simulink model "rev2_PEM"  (R2024a)
settings: Solver=VariableStepAuto  StartTime=0.0  StopTime=10.0  RelTol=1e-3
libraries: spsParallelRLCBranchLib x3, spsControlledVoltageSourceLib x1, spsDiodeLib x1
settings Model: Creator=ADMIN  LastModifiedBy=ADMIN

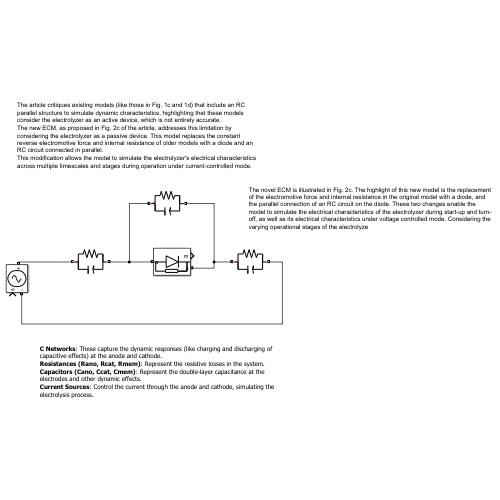
[thumbnail: Simulink's stored preview of the top-level diagram]
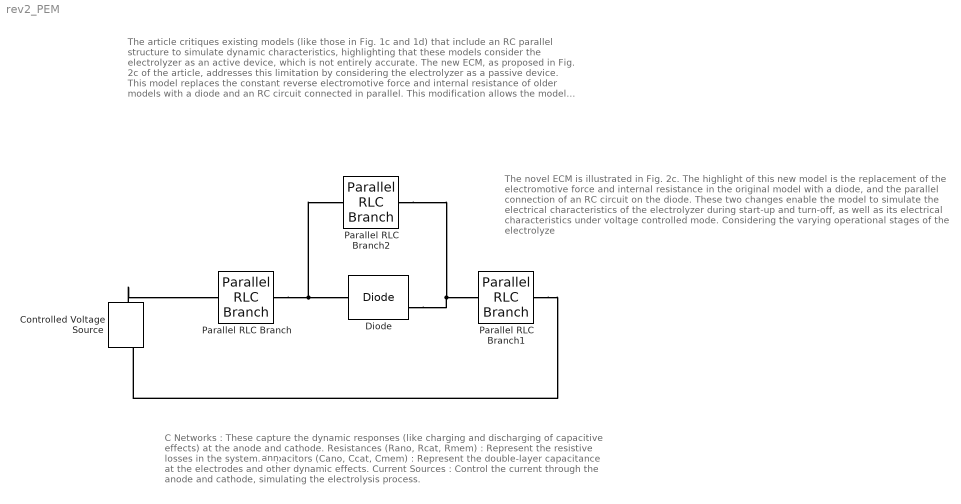
== system rev2_PEM ==
  note: The novel ECM is illustrated in Fig. 2c. The highlight of this new model is the replacement of the electromotive force and internal resistance in the original model with a diode, and the parallel connection of an RC circuit on the diode. These two changes enable the model to simulate the electrical characteristics of the electrolyzer during start-up and turn-off, as well as its electrical characteristics under voltage controlled mode. Considering the varying operational stages of the electrolyze
  note: C Networks : These capture the dynamic responses (like charging and discharging of capacitive effects) at the anode and cathode.
      | Resistances (Rano, Rcat, Rmem) : Represent the resistive losses in the system.
      | Capacitors (Cano, Ccat, Cmem) : Represent the double-layer capacitance at the electrodes and other dynamic effects.
      | Current Sources : Control the current through the anode and cathode, simulating the electrolysis process.
  note: ann
  note: The article critiques existing models (like those in Fig. 1c and 1d) that include an RC parallel structure to simulate dynamic characteristics, highlighting that these models consider the electrolyzer as an active device, which is not entirely accurate.
      | The new ECM, as proposed in Fig. 2c of the article, addresses this limitation by considering the electrolyzer as a passive device. This model replaces the constant reverse electromotive force and internal resistance of older models with a diode and an RC circuit connected in parallel.
      | This modification allows the model to simulate the electrolyzer's electrical characteristics across multiple timescales and stages during operation under current-controlled mode.
  Controlled Voltage Source : spsControlledVoltageSourceLib/Controlled Voltage Source  Initialize=on  Source_Type=AC  Amplitude=0  Phase=0  Frequency=0  Measurements=None
  Diode : spsDiodeLib/Diode  Ron=0.001  Lon=0  Vf=0.8  IC=0  UseSnubber=0  Rs=500  Cs=250e-9  Measurements=on
  Parallel RLC Branch : spsParallelRLCBranchLib/Parallel RLC Branch  LConnTagsString=a  RConnTagsString=__new0  BranchType=RC  Resistance=1  Inductance=1e-3  SetiL0=off  InitialCurrent=0  Capacitance=1e-6  Setx0=off  InitialVoltage=0  Measurements=None
  Parallel RLC Branch1 : spsParallelRLCBranchLib/Parallel RLC Branch  LConnTagsString=a  RConnTagsString=__new0  BranchType=RC  Resistance=1  Inductance=1e-3  SetiL0=off  InitialCurrent=0  Capacitance=1e-6  Setx0=off  InitialVoltage=0  Measurements=None
  Parallel RLC Branch2 : spsParallelRLCBranchLib/Parallel RLC Branch  LConnTagsString=a  RConnTagsString=__new0  BranchType=RC  Resistance=1  Inductance=1e-3  SetiL0=off  InitialCurrent=0  Capacitance=1e-6  Setx0=off  InitialVoltage=0  Measurements=None
  connections:
  Parallel RLC Branch/RConn1 -- Diode/LConn1 -- Parallel RLC Branch2/LConn1
  Parallel RLC Branch2/RConn1 -- Diode/RConn1 -- Parallel RLC Branch1/LConn1
  Controlled Voltage Source/RConn1 -- Parallel RLC Branch/LConn1
  Parallel RLC Branch1/RConn1 -- Controlled Voltage Source/LConn1
